simulink model "gravityGradientTorq"  (R2017a)
settings: Solver=VariableStepAuto  StartTime=0.0  StopTime=10.0  RelTol=1e-3
settings Model: Creator=manoj  LastModifiedBy=manoj

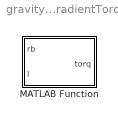
== system gravityGradientTorq ==
  MATLAB Function : MATLAB Function  TreatAsAtomicUnit=on

== matlab function gravityGradientTorq/MATLAB Function ==
  data: rb input; torq output; I input
function torq = fcn(rb,I)
mu=
torq=3*mu/r^5*cross(rb,I*rb)
